simulink model "Elevator_Incorrect_abrir_puerta_Xanet2"  (R2022b)
settings: Solver=VariableStepAuto  StartTime=0.0  StopTime=10.0  RelTol=1e-3
settings Model: Creator=mugarte  LastModifiedBy=Pablo
settings OptimizationCC: ReuseModelBlockBuffer=on

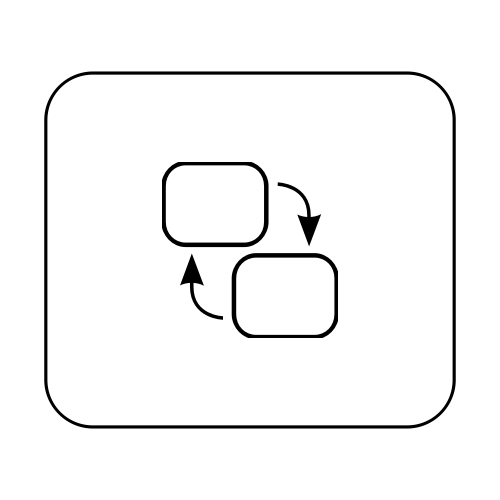
[thumbnail: Simulink's stored preview of the top-level diagram]
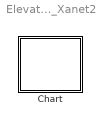
== system Elevator_Incorrect_abrir_puerta_Xanet2 ==
  Chart : Stateflow chart  TreatAsAtomicUnit=on

== stateflow chart Elevator_Incorrect_abrir_puerta_Xanet2/Chart ==
  state Geldirik
    entry:
    atea_kontrola=0;
    abiadura=0;
    pisua_out=oraingoPisua;
  state ateak_ixten
    entry:
    atea_kontrola=-1;
    exit:
    atea_kontrola=0;
  state igotzen
    entry:
    abiadura=15;
    pisua_out=oraingoPisua;
  state jaisten
    entry:
    abiadura = 10;
    pisua_out=oraingoPisua;
    exit:
    atea_kontrola=1;
  state ateak_irekitzen
    entry:
    abiadura=0;
    atea_kontrola=1;
  (default) -> Geldirik : {oraingoPisua=0;}
  ateak_irekitzen -> Geldirik : after(3,sec)
  Geldirik -> ateak_ixten : [pisua~=oraingoPisua]
  ateak_ixten -> (junction 33) : [after(3,sec)]
  (junction 33) -> (junction 39) [order 2] : [pisua<oraingoPisua]
  (junction 33) -> (junction 36) [order 1] : [pisua>oraingoPisua]
  (junction 39) -> jaisten
  (junction 36) -> igotzen
  jaisten -> jaisten [order 2] : after(5, sec){oraingoPisua = oraingoPisua - 1;}
  igotzen -> igotzen [order 2] : after(10, sec){oraingoPisua = oraingoPisua + 1;
      | }
  jaisten -> ateak_irekitzen [order 1] : [pisua==oraingoPisua]
  igotzen -> ateak_irekitzen [order 1] : [pisua==oraingoPisua]
